simulink model "master_task"  (Simulink 7.1)
libraries: mathlib x12
settings Model: Creator=jsobota  LastModifiedBy=jsobota  ExtModeTrigMode=oneshot  ExtModeArmWhenConnect=off

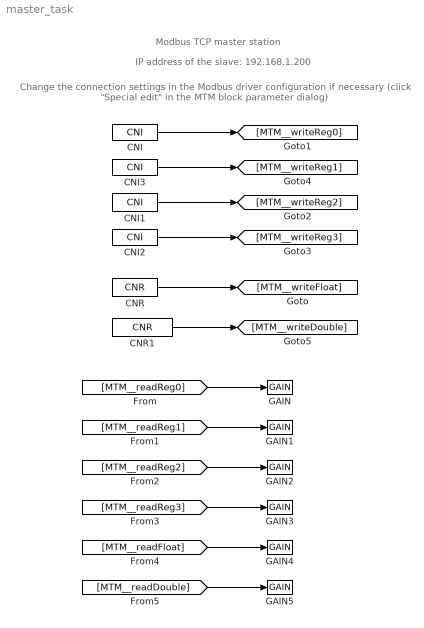
== system master_task ==
  note: Change the connection settings in the Modbus driver configuration
      | if necessary (click "Special edit" in the MTM block parameter dialog)
  note: Modbus TCP master station
  note: IP address of the slave: 192.168.1.200
  CNI : mathlib/CNI  icn=111
  CNI1 : mathlib/CNI  icn=64917
  CNI2 : mathlib/CNI  icn=-29999
  CNI3 : mathlib/CNI  icn=-95
  CNR : mathlib/CNR  ycn=-78.57
  CNR1 : mathlib/CNR  ycn=-79315.18
  GAIN{,1..5} (6 alike) : mathlib/GAIN  k=1
  wires:
  CNI/1 -> [MTM__writeReg0]
  CNI1/1 -> [MTM__writeReg2]
  CNI2/1 -> [MTM__writeReg3]
  CNI3/1 -> [MTM__writeReg1]
  CNR/1 -> [MTM__writeFloat]
  CNR1/1 -> [MTM__writeDouble]
  [MTM__readReg0] -> GAIN/1
  [MTM__readReg1] -> GAIN1/1
  [MTM__readReg2] -> GAIN2/1
  [MTM__readReg3] -> GAIN3/1
  [MTM__readFloat] -> GAIN4/1
  [MTM__readDouble] -> GAIN5/1
